simulink model "observateur_lin_commande_lin"  (R2020a)
settings: Solver=VariableStepAuto  StartTime=0.0  StopTime=100  RelTol=1e-3
undefined symbols (not defined in the file): a, b, K, L_d_lin, L_lin
settings Model: Creator=lenovo  LastModifiedBy=lenovo

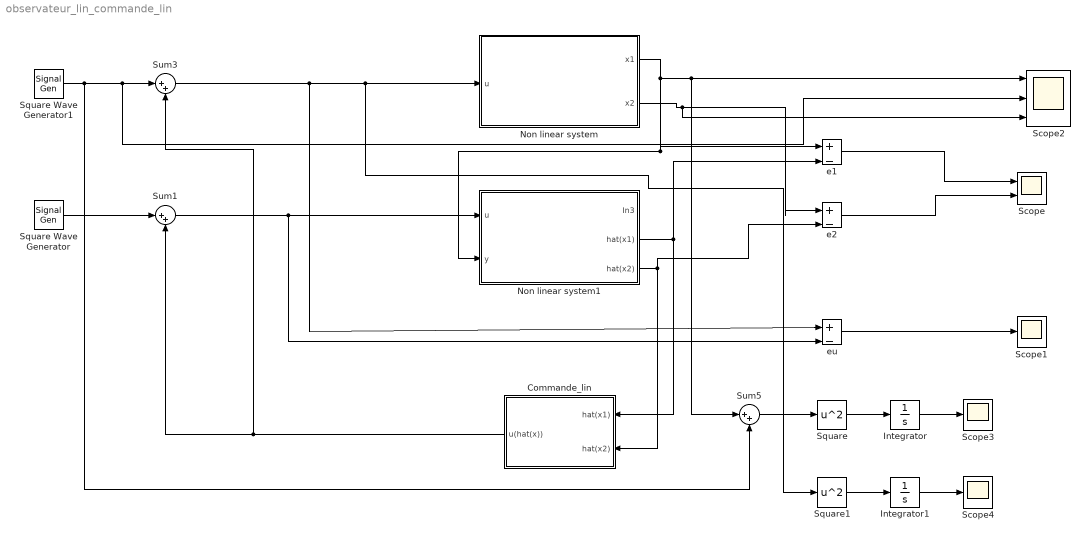
== system observateur_lin_commande_lin ==
  Commande_lin : Subsystem
  Integrator : Integrator
  Integrator1 : Integrator
  Non linear system : Subsystem
  Non linear system1 : Subsystem
      settings: PortSchema="{\"entries\":[{\"content\":{\"sides\":[{\"content\":{\"connectorIds\":[\"In1\",\"In2\"]},\"type\":\"ConnectorPlacement.EquallySpacedRectSide\",\"uuid\":\"618d0c69-a2b8-4648-b070-1c0623f9788f\"},{\"content\":{\"connectorIds\":[\"In3\",\"Out1\",\"Out2\"],\"side\":\"RIGHT\"},\"type\":\"ConnectorPlacement.EquallySpacedRectSide\",\"uuid\":\"79cec027-d132-4f78-855a-d4abd2a9ad58\"},{\"content\":{\"connectorIds\":[],\"side\":\"TOP\"},\"type\":\"ConnectorPlacement.EquallySpacedRectSide\",\"uuid\":\"fcaca530-4b1c-4160-aa00-29a0511fe52c\"}]},\"type\":\"ConnectorPlacement.EquallySpacedConnector\",\"uuid\":\"4273506c-2edc-4fc7-8650-3a7d19e65b58\"}],\"packageUris\":[\"http://schema.mathworks.com/mf0/Connector/19700101\"],\"version\":\"1.0\"}"
  Scope : Scope  NumInputPorts=2
  Scope1 : Scope
  Scope2 : Scope  NumInputPorts=3
  Scope3 : Scope
  Scope4 : Scope
  Square : Math  Operator=square  SaturateOnIntegerOverflow=on
  Square Wave Generator : SignalGenerator  WaveForm=square  Frequency=0.1  Units=rad/sec
  Square Wave Generator1 : SignalGenerator  WaveForm=square  Frequency=0.1  Units=rad/sec
  Square1 : Math  Operator=square  SaturateOnIntegerOverflow=on
  Sum1 : Sum  Inputs=|++
  Sum3 : Sum  Inputs=|++
  Sum5 : Sum  Inputs=|++
  e1 : Sum  Inputs=|+-
  e2 : Sum  Inputs=|+-
  eu : Sum  Inputs=|+-
  wires:
  Non linear system1/2(hat(x2)) -> e2/2, Commande_lin/2(hat(x2))
  Commande_lin/1(u(hat(x))) -> Sum3/2, Sum1/2
  Non linear system1/1(hat(x1)) -> e1/2, Commande_lin/1(hat(x1))
  Sum1/1 -> eu/2, Non linear system1/1(u)
  e2/1 -> Scope/2
  Square Wave Generator/1 -> Sum1/1
  e1/1 -> Scope/1
  eu/1 -> Scope1/1
  Non linear system/1(x1) -> Non linear system1/2(y), e1/1, Sum5/1, Scope2/1
  Non linear system/2(x2) -> Scope2/3, e2/1
  Integrator1/1 -> Scope4/1
  Integrator/1 -> Scope3/1
  Sum3/1 -> eu/1, Square1/1, Non linear system/1(u)
  Square1/1 -> Integrator1/1
  Square Wave Generator1/1 -> Sum5/2, Scope2/2, Sum3/1
  Sum5/1 -> Square/1
  Square/1 -> Integrator/1

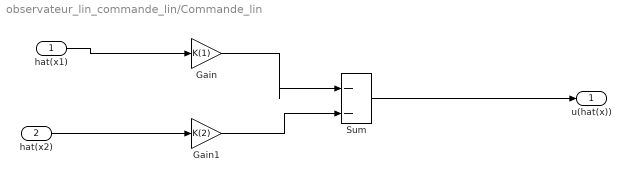
== system observateur_lin_commande_lin/Commande_lin ==
  hat(x1) : Inport
  hat(x2) : Inport  Port=2
  Gain : Gain  Gain=K(1)
  Gain1 : Gain  Gain=K(2)
  Sum : Sum  Inputs=|--
  u(hat(x)) : Outport
  wires:
  Sum/1 -> u(hat(x))/1
  hat(x2)/1 -> Gain1/1
  Gain/1 -> Sum/1
  hat(x1)/1 -> Gain/1
  Gain1/1 -> Sum/2

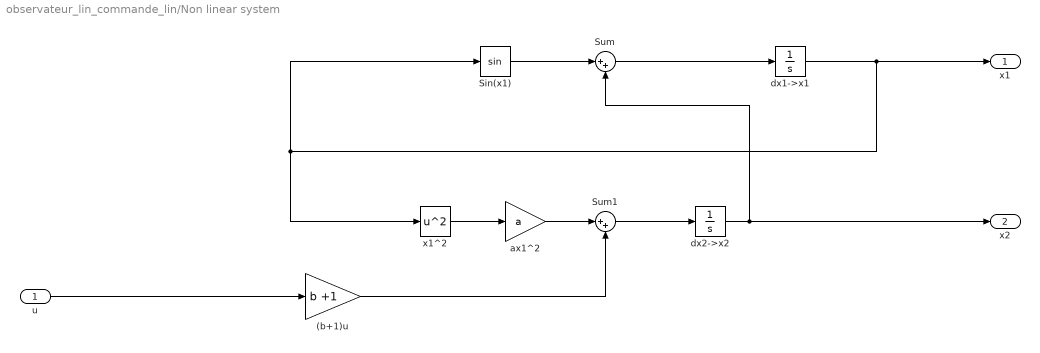
== system observateur_lin_commande_lin/Non linear system ==
  u : Inport
  (b+1)u : Gain  Gain=b +1
  Sin(x1) : Trigonometry
  Sum : Sum  Inputs=|++
  Sum1 : Sum  Inputs=|++
  ax1^2 : Gain  Gain=a
  dx1->x1 : Integrator
  dx2->x2 : Integrator
  x1^2 : Math  Operator=square  SaturateOnIntegerOverflow=on
  x1 : Outport
  x2 : Outport  Port=2
  wires:
  (b+1)u/1 -> Sum1/2
  dx2->x2/1 -> x2/1, Sum/2
  u/1 -> (b+1)u/1
  ax1^2/1 -> Sum1/1
  dx1->x1/1 -> Sin(x1)/1, x1^2/1, x1/1
  Sin(x1)/1 -> Sum/1
  x1^2/1 -> ax1^2/1
  Sum1/1 -> dx2->x2/1
  Sum/1 -> dx1->x1/1

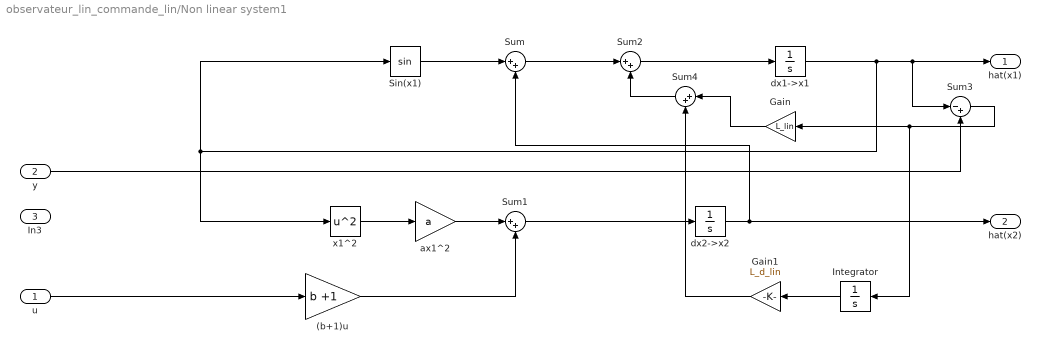
== system observateur_lin_commande_lin/Non linear system1 ==
  u : Inport
  y : Inport  Port=2
  In3 : Inport  Port=3
  (b+1)u : Gain  Gain=b +1
  Gain : Gain  Gain=L_lin
  Gain1 : Gain  Gain=L_d_lin
  Integrator : Integrator
  Sin(x1) : Trigonometry
  Sum{,1..2,4} (4 alike) : Sum  Inputs=|++
  Sum3 : Sum  Inputs=|-+
  ax1^2 : Gain  Gain=a
  dx1->x1 : Integrator
  dx2->x2 : Integrator  InitialCondition=1
  x1^2 : Math  Operator=square  SaturateOnIntegerOverflow=on
  hat(x1) : Outport
  hat(x2) : Outport  Port=2
  wires:
  (b+1)u/1 -> Sum1/2
  dx2->x2/1 -> hat(x2)/1, Sum/2
  u/1 -> (b+1)u/1
  ax1^2/1 -> Sum1/1
  dx1->x1/1 -> Sin(x1)/1, x1^2/1, Sum3/1, hat(x1)/1
  Sin(x1)/1 -> Sum/1
  x1^2/1 -> ax1^2/1
  Sum1/1 -> dx2->x2/1
  y/1 -> Sum3/2
  Sum2/1 -> dx1->x1/1
  Sum/1 -> Sum2/1
  Sum3/1 -> Integrator/1, Gain/1
  Sum4/1 -> Sum2/2
  Gain/1 -> Sum4/1
  Integrator/1 -> Gain1/1
  Gain1/1 -> Sum4/2
